simulink model "my_stateflow"  (R2020a)
settings: Solver=FixedStepDiscrete  StartTime=0.0  StopTime=inf  FixedStep=0.01  RelTol=1e-3
settings Model: Creator=hwh  LastModifiedBy=hwh
settings OptimizationCC: DefaultParameterBehavior=Inlined  EnhancedBackFolding=on  PassReuseOutputArgsAs=Individual arguments  ZeroExternalMemoryAtStartup=off  ZeroInternalMemoryAtStartup=off  OptimizeBlockOrder=speed  DifferentSizesBufferReuse=on  OptimizationCustomize=off  EfficientTunableParamExpr=on
settings DebuggingCC: ParameterTunabilityLossMsg=error
settings SFSimCC: SimCustomHeaderCode="#include \"sf_fsm.h\""  SimUserSources=sf_fsm.c  MATLABDynamicMemAlloc=off
settings SFSimCC: SimUserIncludeDirs=|
  | "..\src";
  | "..\include"
settings RTWCC: SystemTargetFile=ert.tlc  GenCodeOnly=on  TemplateMakefile=ert_default_tmf  GenerateReport=on  RTWUseSimCustomCode=on  CustomHeaderCode="#include \"sf_fsm.h\""  CustomSource=sf_fsm.c  LaunchReport=on
settings RTWCC: CustomInclude=|
  | "..\src";
  | "..\include"
settings CodeAppCC: ForceParamTrailComments=on  IgnoreCustomStorageClasses=off  OperatorAnnotations=on  SimulinkDataObjDesc=on  SFDataObjDesc=on  InsertBlockDesc=on
settings ERTTargetCC: TargetLangStandard=C99 (ISO)  GenerateSampleERTMain=on  InlinedParameterPlacement=NonHierarchical  ERTCustomFileTemplate=example_file_process.tlc

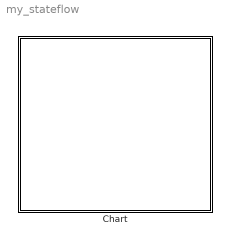
== system my_stateflow ==
  Chart : Stateflow chart  TreatAsAtomicUnit=on

== stateflow chart my_stateflow/Chart ==
  state D [group]
    state High_speed
      en:
      g_msg_out.CurState = state_D_high;
      du:
      g_msg_out.acc = acc_update(state_D_high);
    state Low_speed
      en:
      g_msg_out.CurState = state_D_low;
      du:
      g_msg_out.acc = acc_update(state_D_low);
    state Mid_speed
      en:
      g_msg_out.CurState = state_D_mid;
      du:
      g_msg_out.acc = acc_update(state_D_mid);
    Mid_speed -> High_speed [order 1] : [g_msg_in.speed > 50]
        | {g_msg_out.BrakeState = UnLock;}
    Low_speed -> Mid_speed [order 1] : [g_msg_in.speed > 30]
        | {g_msg_out.BrakeState = UnLock;}
    High_speed -> Mid_speed [order 1] : [g_msg_in.speed < 45]
        | {g_msg_out.BrakeState = UnLock;}
    Mid_speed -> Low_speed [order 2] : [g_msg_in.speed <25]
        | {g_msg_out.BrakeState = UnLock;}
  state P
    en:
    g_msg_out.CurState = state_P;
    du:
    g_msg_out.acc = acc_update(state_P);
  state R
    en:
    g_msg_out.CurState = state_R;
    du:
    g_msg_out.acc = acc_update(state_R);
  Mid_speed -> P [order 3] : [g_msg_in.CarEvent == shift_down]
      | {g_msg_out.BrakeState = BrakeMid;}
  (default) -> P
  P -> Low_speed [order 1] : [g_msg_in.CarEvent == shift_up]
      | {g_msg_out.BrakeState = UnLock;}
  R -> P : [g_msg_in.CarEvent == shift_up]
      | {g_msg_out.BrakeState = BreakReverse;}
  Low_speed -> P [order 2] : [g_msg_in.CarEvent == shift_down]
      | {g_msg_out.BrakeState = BrakeLow;}
  P -> R [order 2] : [g_msg_in.CarEvent == shift_down]
      | {g_msg_out.BrakeState = UnLock;}
  High_speed -> P [order 2] : [g_msg_in.CarEvent == shift_down]
      | {g_msg_out.BrakeState = BrakeHigh;}
